simulink model "rtwdemo_autosar_counter"  (Simulink 7.6)
settings: Solver=FixedStepDiscrete  StartTime=0.0  StopTime=48  FixedStep=0.1  RelTol=1e-3
PreLoadFcn:
  | load rtwdemo_autosar_counter_data;
values from neighbouring files (symbols this model uses):
  LIMIT = Simulink.Parameter    [rtwdemo_international_data.m]
undefined symbols (not defined in the file or in its folder): INC, K, RESET
Description:
  | Algorithm Design
settings Model: Creator=The MathWorks Inc.  ParamWorkspaceSource=ReferencedWorkspace  CovMetricSettings=d  ExtModeTrigMode=oneshot  ExtModeArmWhenConnect=off  ExtModeAutoUpdateStatusClock=off
settings MATStruct: SampleTime=1  Offset=0  Priority=[41.0]
settings DataIOCC: LimitDataPoints=off  SaveFormat=StructureWithTime  SaveOutput=off  SaveTime=off  SignalLoggingName=sigsOut
settings OptimizationCC: InlineParams=on  InlineInvariantSignals=on  StateBitsets=on  DataBitsets=on  UseTempVars=on  ZeroExternalMemoryAtStartup=off  ZeroInternalMemoryAtStartup=off  EfficientFloat2IntCast=on  EfficientMapNaN2IntZero=off  OptimizeModelRefInitCode=on  LifeSpan=1  BufferReusableBoundary=off
settings DebuggingCC: CheckExecutionContextPreStartOutputMsg=on  CheckExecutionContextRuntimeOutputMsg=on  SolverPrmCheckMsg=none  IntegerOverflowMsg=none  StrictBusMsg=ErrorOnBusTreatedAsVector
settings HardwareCC: ProdIntDivRoundTo=Zero  ProdEndianess=LittleEndian  ProdHWDeviceType=Generic->32-bit Embedded Processor  TargetHWDeviceType=Generic->32-bit Embedded Processor
settings ModelReferenceCC: UpdateModelReferenceTargets=IfOutOfDate
settings RTWCC: SystemTargetFile=autosar.tlc  TLCOptions=-p0 -aWarnNonSaturatedBlocks=0  GenCodeOnly=on  TemplateMakefile=ert_default_tmf  Description=AUTOSAR  GenerateReport=on  RTWVerbose=off  ProcessScript=autosar_make_rtw_hook  IncludeHyperlinkInReport=on  LaunchReport=on  GenerateCodeInfo=on
settings CodeAppCC: ForceParamTrailComments=on  IgnoreCustomStorageClasses=off  InsertBlockDesc=on
settings STFCustomTargetCC: ParMdlRefBuildCompliant=on  CompOptLevelCompliant=on  IncludeMdlTerminateFcn=off  CombineOutputUpdateFcns=on  SuppressErrorStatus=on  ERTFirstTimeCompliant=on  ERTCustomFileBanners=on  SupportNonFinite=off  SupportComplex=off  SupportContinuousTime=off  SupportNonInlinedSFcns=off  CPPClassGenCompliant=on  AutosarCompliant=on  SystemTargetFile=autosar.tlc
settings ERTTargetCC: MultiwordLength=2048  IncludeMdlTerminateFcn=off  SuppressErrorStatus=on  SupportNonFinite=off  SupportComplex=off  ModelStepFunctionPrototypeControlCompliant=off  AutosarCompliant=on  ExtModeMexFile=noextcomm  InlinedParameterPlacement=NonHierarchical  ERTCustomFileTemplate=example_file_process.tlc  ERTFilePackagingFormat=CompactWithDataFile  ConvertIfToSwitch=off
settings CustomProperty: DataType=RTWOptions_EnumType__toolbox_rtw_targets_AUTOSAR_AUTOSAR_autosar_1_1AutosarSchemaVersion  Value=3.1
settings EnumStrPairs: String=2.0

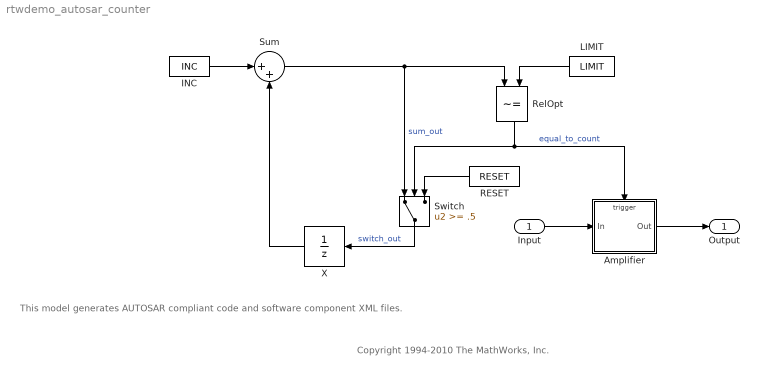
== system rtwdemo_autosar_counter ==
  note: Copyright 1994-2010 The MathWorks, Inc.
  note: This model generates AUTOSAR compliant code and software component XML files.
  Input : Inport  OutDataTypeStr=int32  PortDimensions=1
  Amplifier : Subsystem  TreatAsAtomicUnit=on
  INC : Constant  Description=This block references an AUTOSAR calibration parameter, which is accessed using the AUTOSAR Rte_Calprm function signature.  Value=INC
  LIMIT : Constant  Description=This block references an AUTOSAR calibration parameter, which is accessed using the AUTOSAR Rte_Calprm function signature.  Value=LIMIT
  RESET : Constant  Description=This block references an AUTOSAR calibration parameter, which is accessed using the AUTOSAR Rte_Calprm function signature.  Value=RESET
  RelOpt : RelationalOperator  Operator=~=  InputSameDT=on
  Sum : Sum  Inputs=|++  InputSameDT=on  OutDataTypeStr=Inherit: Same as first input
  Switch : Switch  Threshold=.5  InputSameDT=on
  X : UnitDelay  SampleTime=-1  StateIdentifier=X
  Output : Outport
  wires:
  INC/1 -> Sum/1
  X/1 -> Sum/2
  Switch/1 -> X/1  "switch_out"
  Sum/1 -> Switch/1, RelOpt/1  "sum_out"
  LIMIT/1 -> RelOpt/2
  Input/1 -> Amplifier/1(In)
  RESET/1 -> Switch/3
  RelOpt/1 -> Switch/2, Amplifier/Trigger  "equal_to_count"
  Amplifier/1(Out) -> Output/1

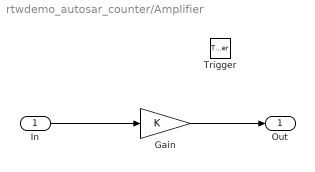
== system rtwdemo_autosar_counter/Amplifier ==
  In : Inport
  Trigger : TriggerPort
  Gain : Gain  Description=This block references an AUTOSAR calibration parameter, which is accessed using the AUTOSAR Rte_Calprm function signature.  Gain=K  OutDataTypeStr=Inherit: Same as input  ParamDataTypeStr=Inherit: Same as input
  Out : Outport  InitialOutput=0
  wires:
  In/1 -> Gain/1
  Gain/1 -> Out/1
